simulink model "Noa_Nofusion_angle"  (R2020b)
settings: Solver=FixedStepDiscrete  StartTime=0.0  StopTime=Inf  FixedStep=0.01  RelTol=1e-3
PostLoadFcn:
  | if any(exist('dsrtsu_mdlpostloadfcn', 'file') ~= 0), dsrtsu_mdlpostloadfcn('Execute', bdroot); end
InitFcn:
  | , if any(exist('rtifpga_mdlclblib', 'file') ~= 0), rtifpga_mdlclblib('Init', bdroot); end,
  | , if any(exist('dsmpb_private', 'file') ~= 0), dsmpb_private('dsmpb_mdlclblib', 'Init', bdroot); end,
undefined symbols (not defined in the file): ACC_TimeGap_DecSetSwt, ACC_TimeGap_IncSetSwt, AccelPedalPosn, AccelPedalPosnVldty, AccelPedlPosnDiagc, AccPedalOverride, ACU_ShiftInProgress, ADAS_Posn_CurLane, AESSwtReq, ALC_SwtReq, BrkPedalSts, CC_ACC_CANCEL_OFFSwt, CC_ACC_CRUISE_OFFSwt, CC_ACC_DecSetSpd_SetSwt, CC_ACC_IncSetSpd_ResuSwt, CC_ACCSwtErr, CharSpd_ms, CSA_NODE, CURRENT_GEAR, CurrentGearValid, DiscIntNeverNeededParam, DrvDoorSts, DrvSBR, DrvTrqReqOvld, ECMACCInterface, ECMRespACC, ELKSwtReq, EngLimpHomeSts, EngSpd, EngState, EngState_PHEV, EngTrqMaxActSpd, EngTrqMinAct, EPS_DrvInpTrqVal_HighReslolution, EPS_FailSts, EPS_LKATorqOvrlDlvd, EPS_LKATorqOvrlDlvdVld, EPS_LKATrqOvlDlvdSts, EPS_SteerMod, EPS_TrqSnsrSts, EQ4_APPINFO, EQ4_LA_ELEM, EQ4_LA_HDR, EQ4_LAP_ELEM, EQ4_LAP_HDR, EQ4_LH_ELEM, EQ4_LH_HDR, EQ4_LRE_ELEM, EQ4_LRE_HDR, ESS_PedSwtReq, ESS_VehSwtReq, FFogLmpSts_F_Pbox, FLWheelDriveDirection, FLWheelSpd, FrntWiprSwtSts, FrntWshrSwtSts, FRWheelDriveDirection, FRWheelSpd, HazardLmpSwtSts, HCU_AccelPedalPosn_Diag ... (+151)
libraries: simulink x138, dsmpblib x33, canfdmsglib x10
(part 13 of 17)

== system Noa_Nofusion_angle/TOS/Subsystem1/ACCOSM/ObjMatrixTransit/Subsystem/For Each Subsystem ==
  <EQ4_OBJ_ELEM> : Inport  Partition=on  PartitionDimension=1  PartitionWidth=1  PartitionOffset=0
  Bus Selector : BusSelector  OutputSignals=OBJ_ID,OBJ_Existence_Probability,OBJ_Object_Class,OBJ_Width,OBJ_Long_Distance,OBJ_Lat_Distance,OBJ_Abs_Long_Acc,OBJ_Abs_Long_Velocity,OBJ_Abs_Lat_Velocity,OBJ_Brake_Light,OBJ_Object_Age,OBJ_Motion_Status,OBJ_Motion_Category,OBJ_Motion_Orientation
  For Each : ForEach  DisableCoverage=on
  id : Outport  ConcatenationDimension=1
  confidence : Outport  Port=2  ConcatenationDimension=1
  classification : Outport  Port=3  ConcatenationDimension=1
  width : Outport  Port=4  ConcatenationDimension=1
  LongDis : Outport  Port=5  ConcatenationDimension=1
  LatDis : Outport  Port=6  ConcatenationDimension=1
  AbsLongAcc : Outport  Port=7  ConcatenationDimension=1
  AbsLongVel : Outport  Port=8  ConcatenationDimension=1
  AbsLatVel : Outport  Port=9  ConcatenationDimension=1
  BrakeLight : Outport  Port=10  ConcatenationDimension=1
  Age : Outport  Port=11  ConcatenationDimension=1
  motionSts : Outport  Port=12  ConcatenationDimension=1
  motionCategory : Outport  Port=13  ConcatenationDimension=1
  motionOrientation : Outport  Port=14  ConcatenationDimension=1
  wires:
  <EQ4_OBJ_ELEM>/1 -> Bus Selector/1
  Bus Selector/12 -> motionSts/1  "<OBJ_Motion_Status>"
  Bus Selector/6 -> LatDis/1  "<OBJ_Lat_Distance>"
  Bus Selector/9 -> AbsLatVel/1  "<OBJ_Abs_Lat_Velocity>"
  Bus Selector/7 -> AbsLongAcc/1  "<OBJ_Abs_Long_Acc>"
  Bus Selector/1 -> id/1  "<OBJ_ID>"
  Bus Selector/2 -> confidence/1  "<OBJ_Existence_Probability>"
  Bus Selector/10 -> BrakeLight/1  "<OBJ_Brake_Light>"
  Bus Selector/8 -> AbsLongVel/1  "<OBJ_Abs_Long_Velocity>"
  Bus Selector/5 -> LongDis/1  "<OBJ_Long_Distance>"
  Bus Selector/11 -> Age/1  "<OBJ_Object_Age>"
  Bus Selector/4 -> width/1  "<OBJ_Width>"
  Bus Selector/14 -> motionOrientation/1  "<OBJ_Motion_Orientation>"
  Bus Selector/3 -> classification/1  "<OBJ_Object_Class>"
  Bus Selector/13 -> motionCategory/1  "<OBJ_Motion_Category>"

== system Noa_Nofusion_angle/TOS/Subsystem1/ACCOSM/ObjMatrixTransit/Subsystem/For Iterator Subsystem ==
  <EQ4_OBJ_ELEM> : Inport
  Bus Selector : BusSelector  OutputSignals=OBJ_ID,OBJ_Existence_Probability,OBJ_Object_Class,OBJ_Width,OBJ_Long_Distance,OBJ_Lat_Distance,OBJ_Abs_Long_Acc,OBJ_Abs_Long_Velocity,OBJ_Abs_Lat_Velocity,OBJ_Brake_Light,OBJ_Object_Age,OBJ_Motion_Status,OBJ_Motion_Category,OBJ_Motion_Orientation
  For Iterator : ForIterator  IterationLimit=20
  Selector : Selector  InputPortWidth=20  IndexOptions=Index vector (port)  Indices=[1 3]  OutputSizes=1
  id : Outport
  confidence : Outport  Port=2
  classification : Outport  Port=3
  width : Outport  Port=4
  LongDis : Outport  Port=5
  LatDis : Outport  Port=6
  AbsLongAcc : Outport  Port=7
  AbsLongVel : Outport  Port=8
  AbsLatVel : Outport  Port=9
  BrakeLight : Outport  Port=10
  Age : Outport  Port=11
  motionSts : Outport  Port=12
  motionCategory : Outport  Port=13
  motionOrientation : Outport  Port=14
  wires:
  <EQ4_OBJ_ELEM>/1 -> Selector/1
  For Iterator/1 -> Selector/2
  Selector/1 -> Bus Selector/1
  Bus Selector/1 -> id/1  "<OBJ_ID>"
  Bus Selector/2 -> confidence/1  "<OBJ_Existence_Probability>"
  Bus Selector/3 -> classification/1  "<OBJ_Object_Class>"
  Bus Selector/4 -> width/1  "<OBJ_Width>"
  Bus Selector/5 -> LongDis/1  "<OBJ_Long_Distance>"
  Bus Selector/6 -> LatDis/1  "<OBJ_Lat_Distance>"
  Bus Selector/7 -> AbsLongAcc/1  "<OBJ_Abs_Long_Acc>"
  Bus Selector/8 -> AbsLongVel/1  "<OBJ_Abs_Long_Velocity>"
  Bus Selector/9 -> AbsLatVel/1  "<OBJ_Abs_Lat_Velocity>"
  Bus Selector/10 -> BrakeLight/1  "<OBJ_Brake_Light>"
  Bus Selector/11 -> Age/1  "<OBJ_Object_Age>"
  Bus Selector/12 -> motionSts/1  "<OBJ_Motion_Status>"
  Bus Selector/13 -> motionCategory/1  "<OBJ_Motion_Category>"
  Bus Selector/14 -> motionOrientation/1  "<OBJ_Motion_Orientation>"

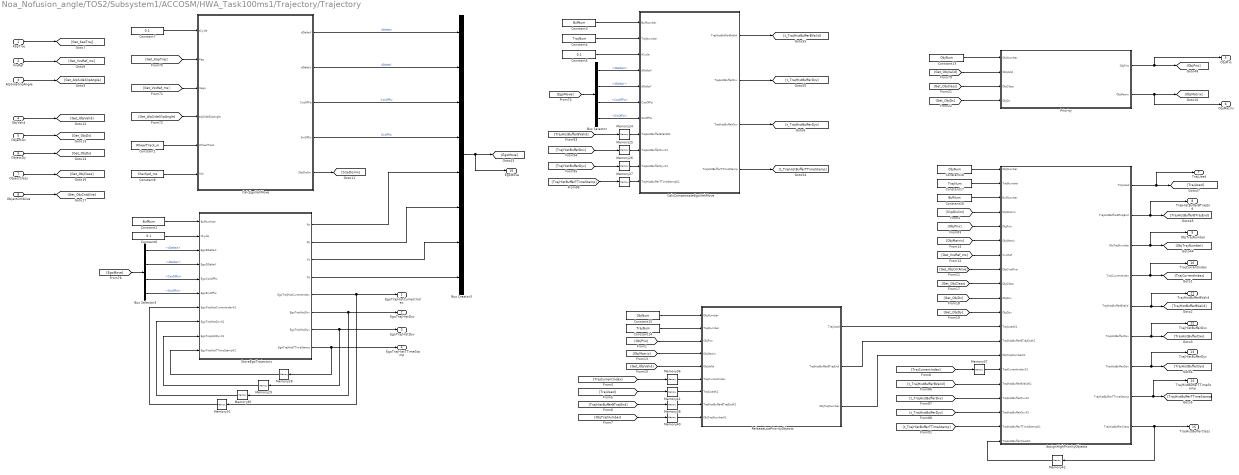
== system Noa_Nofusion_angle/TOS2/Subsystem1/ACCOSM/HWA_Task100ms1/Trajectory/Trajectory ==
  KapTraj : Inport
  VxvRef : Inport  Port=2
  AlpSideSlipAngle : Inport  Port=3
  ObjValid : Inport  Port=4
  ObjectDx : Inport  Port=5
  ObjectDy : Inport  Port=6
  ObjectClass : Inport  Port=7
  ObjectCntAlive : Inport  Port=8
  AssignHighPriorityObjects : MATLAB Function  TreatAsAtomicUnit=on
  Bus Creator3 : BusCreator  Inputs=8
  Bus Selector : BusSelector  OutputSignals=dDeltaX,dDeltaY,CosOfPsi,SinOfPsi
  Bus Selector3 : BusSelector  OutputSignals=dDeltaX,dDeltaY,CosOfPsi,SinOfPsi
  CalcCompensateEgoVehMove : MATLAB Function  TreatAsAtomicUnit=on
  CalcEgoVehMove : MATLAB Function  TreatAsAtomicUnit=on
  Constant1 : Constant  Value=WheelTrack_m  OutDataTypeStr=single
  Constant13 : Constant  Value=ObjNum  OutDataTypeStr=uint8
  Constant14 : Constant  Value=TrajNum  OutDataTypeStr=uint8
  Constant15 : Constant  Value=ObjNum  OutDataTypeStr=uint8
  Constant16 : Constant  Value=BufNum  OutDataTypeStr=uint8
  Constant17 : Constant  Value=TrajNum  OutDataTypeStr=uint8
  Constant18 : Constant  Value=ObjNum  OutDataTypeStr=uint8
  Constant2 : Constant  Value=BufNum  OutDataTypeStr=uint8
  Constant3 : Constant  Value=BufNum  OutDataTypeStr=uint8
  Constant4 : Constant  Value=TrajNum  OutDataTypeStr=uint8
  Constant5 : Constant  Value=0.1  OutDataTypeStr=single
  Constant6 : Constant  Value=0.1  OutDataTypeStr=single
  Constant7 : Constant  Value=0.1  OutDataTypeStr=single
  Constant8 : Constant  Value=CharSpd_ms  OutDataTypeStr=single
  Memory{24..26,42} (4 alike) : Memory  InitialCondition=zeros(TrajNum,BufNum)  InheritSampleTime=on
  Memory27 : Memory  InitialCondition=32*ones(TrajNum,BufNum)  InheritSampleTime=on
  Memory28 : Memory  InitialCondition=32*ones(BufNum,1)  InheritSampleTime=on
  Memory29 : Memory  InitialCondition=zeros(BufNum,1)  InheritSampleTime=on
  Memory30 : Memory  InitialCondition=zeros(BufNum,1)  InheritSampleTime=on
  Memory31 : Memory  InitialCondition=1  InheritSampleTime=on
  Memory36 : Memory  InitialCondition=ones(TrajNum,1)  InheritSampleTime=on
  Memory37 : Memory  InitialCondition=ones(TrajNum,1)  InheritSampleTime=on
  Memory38 : Memory  InitialCondition=ones(TrajNum,BufNum)  InheritSampleTime=on
  Memory40 : Memory  InitialCondition=255*ones(ObjNum,1)  InheritSampleTime=on
  Memory41 : Memory  InitialCondition=zeros(TrajNum,1)  InheritSampleTime=on
  Priority : MATLAB Function  TreatAsAtomicUnit=on
  ReleaseLowPriorityObjects : MATLAB Function  TreatAsAtomicUnit=on
  StoreEgoTrajectory : MATLAB Function  TreatAsAtomicUnit=on
  EgoTrajHistCurrentIndex : Outport
  EgoTrajHistDxv : Outport  Port=2
  EgoTrajHistDyv : Outport  Port=3
  EgoTrajHistTTimeStamp : Outport  Port=4
  ObjPrio : Outport  Port=5
  ObjMatrix : Outport  Port=6
  TrajUsed : Outport  Port=7
  TrajHistBufferBTrajEnd : Outport  Port=8
  ObjTrajNumber : Outport  Port=9
  TrajCurrentIndex : Outport  Port=10
  TrajHistBufferBValid : Outport  Port=11
  TrajHistBufferDxv : Outport  Port=12
  TrajHistBufferDyv : Outport  Port=13
  TrajHistBufferTTimeStamp : Outport  Port=14
  TrajHistBufferClass : Outport  Port=15
  EgoMove : Outport  Port=16
  wires:
  Constant7/1 -> CalcEgoVehMove/1(tCycle)
  [Get_VxvRef_ms] -> CalcEgoVehMove/3(Vego)
  [Get_AlpSideSlipAngle] -> CalcEgoVehMove/4(alpSideSlipAngle)
  [Get_KapTraj] -> CalcEgoVehMove/2(Kap)
  Constant5/1 -> CalcCompensateEgoVehMove/3(tCycle)
  Memory24/1 -> CalcCompensateEgoVehMove/8(TrajHistBufferBValidK1)
  Memory25/1 -> CalcCompensateEgoVehMove/9(TrajHistBufferDxvK1)
  Memory26/1 -> CalcCompensateEgoVehMove/10(TrajHistBufferDyvK1)
  Memory27/1 -> CalcCompensateEgoVehMove/11(TrajHistBufferTTimeStampK1)
  [EgoMove] -> Bus Selector/1
  Bus Selector/1 -> CalcCompensateEgoVehMove/4(dDeltaX)  "<dDeltaX>"
  Bus Selector/2 -> CalcCompensateEgoVehMove/5(dDeltaY)  "<dDeltaY>"
  Bus Selector/3 -> CalcCompensateEgoVehMove/6(CosOfPsi)  "<CosOfPsi>"
  Bus Selector/4 -> CalcCompensateEgoVehMove/7(SinOfPsi)  "<SinOfPsi>"
  [EgoMove] -> Bus Selector3/1
  [Get_ObjDx] -> Priority/4(ObjDx)
  [Get_ObjClass] -> Priority/3(ObjClass)
  [Get_ObjValid] -> Priority/2(ObjValid)
  ReleaseLowPriorityObjects/2(TrajHistBufferBTrajEnd) -> AssignHighPriorityObjects/13(TrajHistBufferBTrajEndK1)
  ReleaseLowPriorityObjects/1(TrajUsed) -> AssignHighPriorityObjects/12(TrajUsedK1)
  AssignHighPriorityObjects/3(ObjTrajNumber) -> ObjTrajNumber/1, [ObjTrajNumber]
  ReleaseLowPriorityObjects/3(ObjTrajNumber) -> AssignHighPriorityObjects/14(ObjTrajNumberK1)
  AssignHighPriorityObjects/1(TrajUsed) -> TrajUsed/1, [TrajUsed]
  AssignHighPriorityObjects/2(TrajHistBufferBTrajEnd) -> TrajHistBufferBTrajEnd/1, [TrajHistBufferBTrajEnd]
  AssignHighPriorityObjects/9(TrajHistBufferClass) -> Memory42/1, TrajHistBufferClass/1
  [ObjPrio] -> AssignHighPriorityObjects/5(ObjPrio)
  CalcCompensateEgoVehMove/1(TrajHistBufferBValid) -> [t_TrajHistBufferBValid]
  [t_TrajHistBufferBValid] -> AssignHighPriorityObjects/16(TrajHistBufferBValidK1)
  CalcCompensateEgoVehMove/2(TrajHistBufferDxv) -> [t_TrajHistBufferDxv]
  [t_TrajHistBufferDxv] -> AssignHighPriorityObjects/17(TrajHistBufferDxvK1)
  [t_TrajHistBufferDyv] -> AssignHighPriorityObjects/18(TrajHistBufferDyvK1)
  CalcCompensateEgoVehMove/4(TrajHistBufferTTimeStamp) -> [t_TrajHistBufferTTimeStamp]
  [t_TrajHistBufferTTimeStamp] -> AssignHighPriorityObjects/19(TrajHistBufferTTimeStampK1)
  Memory36/1 -> ReleaseLowPriorityObjects/6(TrajCurrentIndex)
  Memory37/1 -> AssignHighPriorityObjects/15(TrajCurrentIndexK1)
  Memory38/1 -> ReleaseLowPriorityObjects/8(TrajHistBufferBTrajEndK1)
  Memory40/1 -> ReleaseLowPriorityObjects/9(ObjTrajNumberK1)
  Memory41/1 -> ReleaseLowPriorityObjects/7(TrajUsedK1)
  Memory42/1 -> AssignHighPriorityObjects/20(TrajHistBufferClassK1)
  [TrajUsed] -> Memory41/1
  [ObjTrajNumber] -> Memory40/1
  [TrajHistBufferBTrajEnd] -> Memory38/1
  [ObjPrio] -> ReleaseLowPriorityObjects/3(ObjPrio)
  [Get_ObjValid] -> ReleaseLowPriorityObjects/5(ObjValid)
  AssignHighPriorityObjects/5(TrajHistBufferBValid) -> TrajHistBufferBValid/1, [TrajHistBufferBValid]
  AssignHighPriorityObjects/7(TrajHistBufferDyv) -> TrajHistBufferDyv/1, [TrajHistBufferDyv]
  AssignHighPriorityObjects/6(TrajHistBufferDxv) -> TrajHistBufferDxv/1, [TrajHistBufferDxv]
  [TrajCurrentIndex] -> Memory36/1
  [TrajCurrentIndex] -> Memory37/1
  [Get_VxvRef_ms] -> AssignHighPriorityObjects/7(VxvRef)
  [Get_ObjClass] -> AssignHighPriorityObjects/9(ObjClass)
  [Get_ObjDx] -> AssignHighPriorityObjects/10(ObjDxv)
  AssignHighPriorityObjects/4(TrajCurrentIndex) -> TrajCurrentIndex/1, [TrajCurrentIndex]
  [Get_ObjDy] -> AssignHighPriorityObjects/11(ObjDyv)
  [TrajHistBufferTTimeStamp] -> Memory27/1
  [TrajHistBufferDxv] -> Memory25/1
  [TrajHistBufferDyv] -> Memory26/1
  [TrajHistBufferBValid] -> Memory24/1
  [Get_ObjCntAlive] -> AssignHighPriorityObjects/8(ObjCntAlive)
  KapTraj/1 -> [Get_KapTraj]
  VxvRef/1 -> [Get_VxvRef_ms]
  AlpSideSlipAngle/1 -> [Get_AlpSideSlipAngle]
  Constant3/1 -> CalcCompensateEgoVehMove/1(BufNumber)
  Constant4/1 -> CalcCompensateEgoVehMove/2(TrajNumber)
  Constant13/1 -> Priority/1(ObjNumber)
  Constant15/1 -> ReleaseLowPriorityObjects/1(ObjNumber)
  Constant14/1 -> ReleaseLowPriorityObjects/2(TrajNumber)
  Constant18/1 -> AssignHighPriorityObjects/1(ObjNumber)
  Constant17/1 -> AssignHighPriorityObjects/2(TrajNumber)
  Constant16/1 -> AssignHighPriorityObjects/3(BufNumber)
  [ObjMatrix] -> ReleaseLowPriorityObjects/4(ObjMatrix)
  [ObjMatrix] -> AssignHighPriorityObjects/6(ObjMatrix)
  Constant2/1 -> StoreEgoTrajectory/1(BufNumber)
  Constant6/1 -> StoreEgoTrajectory/2(tCycle)
  StoreEgoTrajectory/7(EgoTrajHistDyv) -> EgoTrajHistDyv/1, Memory29/1
  Memory28/1 -> StoreEgoTrajectory/10(EgoTrajHistTTimeStampK1)
  Memory29/1 -> StoreEgoTrajectory/9(EgoTrajHistDyvK1)
  StoreEgoTrajectory/6(EgoTrajHistDxv) -> EgoTrajHistDxv/1, Memory30/1
  Memory30/1 -> StoreEgoTrajectory/8(EgoTrajHistDxvK1)
  StoreEgoTrajectory/5(EgoTrajHistCurrentIndex) -> EgoTrajHistCurrentIndex/1, Memory31/1
  Memory31/1 -> StoreEgoTrajectory/7(EgoTrajHistCurrentIndexK1)
  StoreEgoTrajectory/8(EgoTrajHistTTimeStamp) -> EgoTrajHistTTimeStamp/1, Memory28/1
  Bus Selector3/3 -> StoreEgoTrajectory/5(EgoCosOfPsi)  "<CosOfPsi>"
  Bus Selector3/2 -> StoreEgoTrajectory/4(EgoDDeltaY)  "<dDeltaY>"
  Bus Selector3/4 -> StoreEgoTrajectory/6(EgoSinOfPsi)  "<SinOfPsi>"
  Bus Selector3/1 -> StoreEgoTrajectory/3(EgoDDeltaX)  "<dDeltaX>"
  AssignHighPriorityObjects/8(TrajHistBufferTTimeStamp) -> TrajHistBufferTTimeStamp/1, [TrajHistBufferTTimeStamp]
  ObjValid/1 -> [Get_ObjValid]
  ObjectDy/1 -> [Get_ObjDy]
  ObjectDx/1 -> [Get_ObjDx]
  ObjectClass/1 -> [Get_ObjClass]
  ObjectCntAlive/1 -> [Get_ObjCntAlive]
  CalcEgoVehMove/1(dDeltaX) -> Bus Creator3/1  "dDeltaX"
  CalcEgoVehMove/2(dDeltaY) -> Bus Creator3/2  "dDeltaY"
  CalcEgoVehMove/3(CosOfPsi) -> Bus Creator3/3  "CosOfPsi"
  CalcEgoVehMove/4(SinOfPsi) -> Bus Creator3/4  "SinOfPsi"
  Priority/1(ObjPrio) -> ObjPrio/1, [ObjPrio]
  Priority/2(ObjMatrix) -> [ObjMatrix], ObjMatrix/1
  CalcCompensateEgoVehMove/3(TrajHistBufferDyv) -> [t_TrajHistBufferDyv]
  Constant1/1 -> CalcEgoVehMove/5(WheelTrack)
  Constant8/1 -> CalcEgoVehMove/6(Vch)
  CalcEgoVehMove/5(SlipDislim) -> [SlipDislim]
  [SlipDislim] -> AssignHighPriorityObjects/4(SlipDisLim)
  Bus Creator3/1 -> EgoMove/1, [EgoMove]
  StoreEgoTrajectory/4(Pd) -> Bus Creator3/8
  StoreEgoTrajectory/3(Pc) -> Bus Creator3/7
  StoreEgoTrajectory/2(Pb) -> Bus Creator3/6
  StoreEgoTrajectory/1(Pa) -> Bus Creator3/5

== system Noa_Nofusion_angle/TOS2/Subsystem1/ACCOSM/ObjMatrixTransit/Subsystem/For Each Subsystem ==
  <EQ4_OBJ_ELEM> : Inport  Partition=on  PartitionDimension=1  PartitionWidth=1  PartitionOffset=0
  Bus Selector : BusSelector  OutputSignals=OBJ_ID,OBJ_Existence_Probability,OBJ_Object_Class,OBJ_Width,OBJ_Long_Distance,OBJ_Lat_Distance,OBJ_Abs_Long_Acc,OBJ_Abs_Long_Velocity,OBJ_Abs_Lat_Velocity,OBJ_Brake_Light,OBJ_Object_Age,OBJ_Motion_Status,OBJ_Motion_Category,OBJ_Motion_Orientation
  For Each : ForEach  DisableCoverage=on
  id : Outport  ConcatenationDimension=1
  confidence : Outport  Port=2  ConcatenationDimension=1
  classification : Outport  Port=3  ConcatenationDimension=1
  width : Outport  Port=4  ConcatenationDimension=1
  LongDis : Outport  Port=5  ConcatenationDimension=1
  LatDis : Outport  Port=6  ConcatenationDimension=1
  AbsLongAcc : Outport  Port=7  ConcatenationDimension=1
  AbsLongVel : Outport  Port=8  ConcatenationDimension=1
  AbsLatVel : Outport  Port=9  ConcatenationDimension=1
  BrakeLight : Outport  Port=10  ConcatenationDimension=1
  Age : Outport  Port=11  ConcatenationDimension=1
  motionSts : Outport  Port=12  ConcatenationDimension=1
  motionCategory : Outport  Port=13  ConcatenationDimension=1
  motionOrientation : Outport  Port=14  ConcatenationDimension=1
  wires:
  <EQ4_OBJ_ELEM>/1 -> Bus Selector/1
  Bus Selector/12 -> motionSts/1  "<OBJ_Motion_Status>"
  Bus Selector/6 -> LatDis/1  "<OBJ_Lat_Distance>"
  Bus Selector/9 -> AbsLatVel/1  "<OBJ_Abs_Lat_Velocity>"
  Bus Selector/7 -> AbsLongAcc/1  "<OBJ_Abs_Long_Acc>"
  Bus Selector/1 -> id/1  "<OBJ_ID>"
  Bus Selector/2 -> confidence/1  "<OBJ_Existence_Probability>"
  Bus Selector/10 -> BrakeLight/1  "<OBJ_Brake_Light>"
  Bus Selector/8 -> AbsLongVel/1  "<OBJ_Abs_Long_Velocity>"
  Bus Selector/5 -> LongDis/1  "<OBJ_Long_Distance>"
  Bus Selector/11 -> Age/1  "<OBJ_Object_Age>"
  Bus Selector/4 -> width/1  "<OBJ_Width>"
  Bus Selector/14 -> motionOrientation/1  "<OBJ_Motion_Orientation>"
  Bus Selector/3 -> classification/1  "<OBJ_Object_Class>"
  Bus Selector/13 -> motionCategory/1  "<OBJ_Motion_Category>"

== system Noa_Nofusion_angle/TOS2/Subsystem1/ACCOSM/ObjMatrixTransit/Subsystem/For Iterator Subsystem ==
  <EQ4_OBJ_ELEM> : Inport
  Bus Selector : BusSelector  OutputSignals=OBJ_ID,OBJ_Existence_Probability,OBJ_Object_Class,OBJ_Width,OBJ_Long_Distance,OBJ_Lat_Distance,OBJ_Abs_Long_Acc,OBJ_Abs_Long_Velocity,OBJ_Abs_Lat_Velocity,OBJ_Brake_Light,OBJ_Object_Age,OBJ_Motion_Status,OBJ_Motion_Category,OBJ_Motion_Orientation
  For Iterator : ForIterator  IterationLimit=20
  Selector : Selector  InputPortWidth=20  IndexOptions=Index vector (port)  Indices=[1 3]  OutputSizes=1
  id : Outport
  confidence : Outport  Port=2
  classification : Outport  Port=3
  width : Outport  Port=4
  LongDis : Outport  Port=5
  LatDis : Outport  Port=6
  AbsLongAcc : Outport  Port=7
  AbsLongVel : Outport  Port=8
  AbsLatVel : Outport  Port=9
  BrakeLight : Outport  Port=10
  Age : Outport  Port=11
  motionSts : Outport  Port=12
  motionCategory : Outport  Port=13
  motionOrientation : Outport  Port=14
  wires:
  <EQ4_OBJ_ELEM>/1 -> Selector/1
  For Iterator/1 -> Selector/2
  Selector/1 -> Bus Selector/1
  Bus Selector/1 -> id/1  "<OBJ_ID>"
  Bus Selector/2 -> confidence/1  "<OBJ_Existence_Probability>"
  Bus Selector/3 -> classification/1  "<OBJ_Object_Class>"
  Bus Selector/4 -> width/1  "<OBJ_Width>"
  Bus Selector/5 -> LongDis/1  "<OBJ_Long_Distance>"
  Bus Selector/6 -> LatDis/1  "<OBJ_Lat_Distance>"
  Bus Selector/7 -> AbsLongAcc/1  "<OBJ_Abs_Long_Acc>"
  Bus Selector/8 -> AbsLongVel/1  "<OBJ_Abs_Long_Velocity>"
  Bus Selector/9 -> AbsLatVel/1  "<OBJ_Abs_Lat_Velocity>"
  Bus Selector/10 -> BrakeLight/1  "<OBJ_Brake_Light>"
  Bus Selector/11 -> Age/1  "<OBJ_Object_Age>"
  Bus Selector/12 -> motionSts/1  "<OBJ_Motion_Status>"
  Bus Selector/13 -> motionCategory/1  "<OBJ_Motion_Category>"
  Bus Selector/14 -> motionOrientation/1  "<OBJ_Motion_Orientation>"

== matlab function Noa_Nofusion_angle/TOS2/Subsystem1/ACCOSM/HWA_Task100ms1/OTL1/P0TrajHistCalc1 ==
  data: P0TrajHistNum output uint8; P0TrajHistNum1 input uint8; P0TrajHistDxv1 input single; P0TrajHistDxv output single; P0TrajHistDyv1 input single; P0TrajHistDyv output single; LineValid output boolean; a output single; b output single; c output single; d output single; dxMin output single; dxMax output single
function [P0TrajHistNum,P0TrajHistDxv,P0TrajHistDyv,LineValid,a,b,c,d,dxMin,dxMax] = P0TrajHistMixCalc(...
    P0TrajHistNum1,P0TrajHistDxv1,P0TrajHistDyv1)

P0TrajHistDxv = single(zeros(48,1));
P0TrajHistDyv = single(zeros(48,1));
P0TrajHistNum = uint8(0);

if (P0TrajHistNum1>0)
    P0TrajHistDxv(1:P0TrajHistNum1) = P0TrajHistDxv1(1:P0TrajHistNum1);
    P0TrajHistDyv(1:P0TrajHistNum1) = P0TrajHistDyv1(1:P0TrajHistNum1);
    P0TrajHistNum = P0TrajHistNum1;
end

if P0TrajHistNum>=4
    dxMin = P0TrajHistDxv(P0TrajHistNum);
    dxMax = P0TrajHistDxv(1) + 6;
%     q2 = max(ceil(P0TrajHistNum/2),2);
%     q3 = max(ceil(P0TrajHistNum*3/4),3);
%     q4 = P0TrajHistNum;
%     MaX = [P0TrajHistDxv(1);P0TrajHistDxv(q2);P0TrajHistDxv(q3);P0TrajHistDxv(q4)];
%     MaY = [P0TrajHistDyv(1);P0TrajHistDyv(q2);P0TrajHistDyv(q3);P0TrajHistDyv(q4)];
%     [~,b,c,d] = pl(MaX,MaY);
    P = polyfit(P0TrajHistDxv(1:P0TrajHistNum),P0TrajHistDyv(1:P0TrajHistNum),2);
    b = P(1);
    c = P(2);
    d = P(3);

    a = single(0);
   LineValid = true;
   if dxMin>0.5
      LineValid = false; 
   end
else
   dxMin = single(0); 
   dxMax = single(0); 
   a = single(0);
   b = single(0);
   c = single(0);
   d = single(0);
   LineValid = false;
end

== matlab function Noa_Nofusion_angle/TOS2/Subsystem1/ACCOSM/HWA_Task100ms1/Plaus ==
  data: dxMaxFollow input single size=1; ObjValid input boolean size=15; ObjDx input single size=15; ObjVx input single size=15; ObjPlaus output single size=15; ObjOnLeft input single size=15; ObjPlausLeft output single size=15; ObjPlausRight output single size=15; ObjOnRight input single size=15; ObjDycHist input single size=15; ObjqDycHist input single size=15; ObjLpb input single size=15; ObjLpbLeft input single size=15; ObjLpbRight input single size=15; ObjPlausK1 input single size=15; ObjPlausLeftK1 input single size=15; ObjPlausRightK1 input single size=15
function [ObjPlaus,ObjPlausLeft,ObjPlausRight] = ...
    PlausCalc(dxMaxFollow,ObjValid,ObjDx,ObjVx,ObjOnLeft,ObjOnRight,ObjDycHist,ObjqDycHist,...
    ObjLpb,ObjLpbLeft,ObjLpbRight,ObjPlausK1,ObjPlausLeftK1,ObjPlausRightK1)

[ObjPlaus,ObjPlausLeft,ObjPlausRight] = ...
    PlausCalc(dxMaxFollow,ObjValid,ObjDx,ObjVx,ObjOnLeft,ObjOnRight,ObjDycHist,ObjqDycHist,...
    ObjLpb,ObjLpbLeft,ObjLpbRight,ObjPlausK1,ObjPlausLeftK1,ObjPlausRightK1);
end

== matlab function Noa_Nofusion_angle/TOS2/Subsystem1/ACCOSM/HWA_Task100ms1/Spw ==
  data: AlpSumSlideCurveness input single size=1; kapCourseErr input single size=1; ObjSpw output single size=15; ObjValid input boolean size=15; DycASI input single size=15; ObjDx input single size=15; ObjSpwLeft output single size=15; ObjSpwRight output single size=15; ObjOnLeft output; ObjOnRight output; ObjDyc input; ObjDycHist input; ObjqDycHist input; ObjDycASI output; ObjDyKapErr output
function [ObjSpw,ObjSpwLeft,ObjSpwRight,ObjOnLeft,ObjOnRight,ObjDycASI,ObjDyKapErr] = ...
    CalcSpw(AlpSumSlideCurveness,kapCourseErr,ObjValid,DycASI,ObjDx,ObjDyc,ObjDycHist,ObjqDycHist)
 
ObjSpw = single(zeros(15,1));
ObjSpwLeft = single(zeros(15,1));
ObjSpwRight = single(zeros(15,1));
ObjOnLeft = single(zeros(15,1));
ObjOnRight = single(zeros(15,1));
ObjDycASI = single(zeros(15,1));
ObjDyKapErr = single(zeros(15,1));
 
for i=1:15
    if ObjValid(i)
        t_dycASI = DycASI(i);
        t_kapErrMin = single(0.0002);
        t_kapErrCurvenessMax = single(0.0018);
        
        temp1 = min(AlpSumSlideCurveness,single(1));
        t_kapErrCurveness = t_kapErrCurvenessMax*temp1;
        t_kapErr = max(t_kapErrMin,max(kapCourseErr,t_kapErrCurveness));
        temp1 = min(ObjDx(i),single(80));
        t_DyKapErr = t_kapErr*temp1*temp1/2;
        ObjDyKapErr(i) = t_DyKapErr;
        
        %         t_dyHalfLane = 1.5;
        %         t_dy3halfLane = 5.25;
        
        if abs(t_dycASI)>=4.5
            t_spw = single(0);
            t_spwNeighbour = single(0);
        elseif abs(t_dycASI)>=3
            t_spw = single(0);
            t_dycToLane = abs(t_dycASI) - single(3);
            t_spwNeighbour = CalcSPW(t_dycToLane,single(3),t_DyKapErr);
        elseif abs(t_dycASI)>=1.5
            t_spw = single(0);
            t_spwNeighbour = CalcSPW(single(0),single(3),t_DyKapErr);
        else
            t_spwNeighbour = single(0);
            t_spw = CalcSPW(single(0),single(3),t_DyKapErr);
        end
        if t_dycASI>=0
            t_spwRight = single(0);
            t_spwLeft = t_spwNeighbour;
        else
            t_spwLeft = single(0);
            t_spwRight = t_spwNeighbour;
        end
        ObjSpw(i) = t_spw;
        ObjSpwLeft(i) = t_spwLeft;
        ObjSpwRight(i) = t_spwRight;
        % -------------------------------------------------------------------------
        
        temp1 = 0.5*ObjqDycHist(i);
        t_dycASI = ObjDyc(i)*(1-temp1) + ObjDycHist(i)*temp1;
        temp2 = single(1.5) + t_DyKapErr;
        temp3 = single(3) + t_DyKapErr;
        ObjDycASI(i) = t_dycASI;
        
        if t_dycASI>=0
            temp1 = max(single(1.5),min(temp3,t_dycASI)) - single(1.5);
            ObjOnLeft(i) = min(single(1),temp1/temp2);
        else
            temp1 = max(min(single(-1.5),t_dycASI),-temp3);
            temp1 = -temp1 - single(1.5);
            ObjOnRight(i) = min(single(1),temp1/temp2);
        end
    end
end
end
 
function t_spw = CalcSPW(absDyc,dyLaneWidth,dyKapErr)
temp3 = dyLaneWidth/2;
temp1 = temp3 - dyKapErr;
temp2 = temp3 + dyKapErr;
temp2 = min(temp2,dyLaneWidth);
 
if absDyc<=temp1
    t_spw = single(1);
elseif absDyc>=temp2
    t_spw = single(0);
else
    temp3 = temp2 - absDyc;
    temp4 = 2*dyKapErr;
    t_spw = temp3/temp4;
end
end

== matlab function Noa_Nofusion_angle/TOS2/Subsystem1/ACCOSM/HWA_Task100ms1/Std ==
  data: u input; y output
function y = fcn(u)

y = std(u);

== stateflow chart Noa_Nofusion_angle/Common/Subsystem7/DS/DriverSts_StateMachine ==
  state DriverSts [group]
    0x0:DriverUnbeliv
    0x1:DriverGood
    0x2:DriverLowDistractn
    0x3:DriverMidDistractn
    0x4:DriverHi1Distractn
    0x5:DriverHi2Distractn
    0x6:DriverLowDrowsiness
    0x7:DriverMidDrowsiness
    0x8:DriverHi1Drowsiness
    0x9:DriverHi2Drowsiness
  state DistractnSts [group]
    0x0:DMSNoDistractn
    0x1:DMSLowDistractn
    0x2:DMSMidDistractn
    0x3:DMSHi1Distractn
    0x4:DMSHi2Distractn
    0x5:DMSUnbelievDistractn
    DrowsnsSts
    0x0:DMSNoDrowsiness
    0x1:DMSLowDrowsiness
    0x2:DMSMidDrowsiness
    0x3:DMSHi1Drowsiness
    0x4:DMSHi2Drowsiness
    0x5:DMSUnbelievDrowsiness
  state Ini
    entry: DriverSts=DriverUnbeliv;
    DADistractnNoDistractn=0;
    DADrowsnsNoDrowsiness=0;
  state Unbelievable
    entry: DriverSts=DriverUnbeliv;
    DistractnSts=DMSUnbelievDistractn;
    DrowsnsSts=DMSUnbelievDrowsiness;
  state Good
    entry:DriverSts=DriverGood;
    DistractnSts=DMSNoDistractn;
    DrowsnsSts=DMSNoDrowsiness;
  state DDA
    state Distractn [parallel]
      settings: executionOrder=1
      state NoDis
        entry:DistractnSts=DMSNoDistractn;
        DADistractnNoDistractn=1;
        exit:DADistractnNoDistractn=0;
      state ExistDis
        state LowDis
          entry:DistractnSts=DMSLowDistractn;
        state MidDis
          entry:DistractnSts=DMSMidDistractn;
        state Hi1Dis
          entry:DistractnSts=DMSHi1Distractn;
        state Hi2Dis
          entry:DistractnSts=DMSHi2Distractn;
        LowDis -> (junction 143) [order 2] : [DSOther2Hi1Distractn]
        (junction 143) -> (junction 126)
        (default) -> (junction 137)
        (junction 137) -> LowDis [order 1] : [DSGoodUnbeliv2LowDistractn]
        (junction 146) -> LowDis
        (junction 147) -> (junction 146)
        (junction 137) -> (junction 142) [order 2]
        (junction 144) -> (junction 146) [order 1] : [DSMidHi1Hi22LowDistractn]
        (junction 124) -> (junction 147) [order 1] : [DSMidHi1Hi22LowDistractn]
        LowDis -> MidDis [order 1] : [DSLow2MidDistractn]
        MidDis -> LowDis [order 2] : [DSMidHi1Hi22LowDistractn]
        (junction 142) -> MidDis [order 1] : [DSGoodUnbeliv2MidDistractn]
        (junction 144) -> MidDis [order 2]
        (junction 124) -> (junction 144) [order 2]
        (junction 142) -> (junction 138) [order 2]
        Hi2Dis -> (junction 144) : [DSHi1Hi22MidDistractn||......
            | DSMidHi1Hi22LowDistractn]
        (junction 130) -> (junction 124)
        MidDis -> Hi1Dis [order 1] : [DSOther2Hi1Distractn]
        Hi1Dis -> MidDis [order 2] : [DSHi1Hi22MidDistractn]
        Hi1Dis -> Hi2Dis [order 1] : [DSOther2Hi2Distractn]
        (junction 138) -> Hi1Dis
        (junction 126) -> Hi1Dis
        Hi1Dis -> (junction 130) [order 3] : [DSHi1Hi22MidDistractn||......
            | DSMidHi1Hi22LowDistractn]
      (default) -> (junction 122)
      (junction 122) -> NoDis [order 2]
      (junction 122) -> ExistDis [order 1] : [DSGoodUnbeliv2LowDistractn||......
          | DSGoodUnbeliv2MidDistractn||......
          | DSOther2Hi1Distractn]
      NoDis -> ExistDis : [DSGoodUnbeliv2LowDistractn||......
          | DSGoodUnbeliv2MidDistractn||......
          | DSOther2Hi1Distractn]
      ExistDis -> NoDis : [DSMidHi1Hi22NoDistractn]
    state Drowsns [parallel]
      settings: executionOrder=2
      state NoDrow
        entry:DrowsnsSts=DMSNoDrowsiness;
        DADrowsnsNoDrowsiness=1;
        exit:DADrowsnsNoDrowsiness=0;
      state ExistDrow
        state LowDrow
          entry:DrowsnsSts=DMSLowDrowsiness;
        state MidDrow
          entry:DrowsnsSts=DMSMidDrowsiness;
        state Hi1Drow
          entry:DrowsnsSts=DMSHi1Drowsiness;
        state Hi2Drow
          entry:DrowsnsSts=DMSHi2Drowsiness;
        LowDrow -> (junction 58) [order 2] : [DSOther2Hi1Drowsns]
        (junction 58) -> (junction 46)
        (default) -> (junction 36)
        (junction 36) -> LowDrow [order 1] : [DSGoodUnbeliv2LowDrowsns]
        (junction 10) -> LowDrow
        (junction 74) -> (junction 10)
        (junction 36) -> (junction 42) [order 2]
        (junction 11) -> (junction 10) [order 1] : [DSMidHi1Hi22LowDrowsns]
        (junction 61) -> (junction 74) [order 1] : [DSMidHi1Hi22LowDrowsns]
        LowDrow -> MidDrow [order 1] : [DSLow2MidDrowsns]
        MidDrow -> LowDrow [order 2] : [DSMidHi1Hi22LowDrowsns]
        (junction 42) -> MidDrow [order 1] : [DSGoodUnbeliv2MidDrowsns]
        (junction 11) -> MidDrow [order 2]
        (junction 61) -> (junction 11) [order 2]
        (junction 42) -> (junction 59) [order 2]
        Hi2Drow -> (junction 11) : [DSMidHi1Hi22LowDrowsns||......
            | DSHi1Hi22MidDrowsns]
        (junction 39) -> (junction 61)
        MidDrow -> Hi1Drow [order 1] : [DSOther2Hi1Drowsns]
        Hi1Drow -> MidDrow [order 2] : [DSHi1Hi22MidDrowsns]
        Hi1Drow -> Hi2Drow [order 1] : [DSOther2Hi2Drowsns]
        (junction 59) -> Hi1Drow
        (junction 46) -> Hi1Drow
        Hi1Drow -> (junction 39) [order 3] : [DSMidHi1Hi22LowDrowsns||......
            | DSHi1Hi22MidDrowsns]
      (default) -> (junction 72)
      (junction 72) -> NoDrow [order 2]
      (junction 72) -> ExistDrow [order 1] : [DSGoodUnbeliv2LowDrowsns||......
          | DSGoodUnbeliv2MidDrowsns||......
          | DSOther2Hi1Drowsns]
      NoDrow -> ExistDrow : [DSGoodUnbeliv2LowDrowsns||......
          | DSGoodUnbeliv2MidDrowsns||......
          | DSOther2Hi1Drowsns]
      ExistDrow -> NoDrow : [DSMidHi1Hi22NoDrowsns]
    state Arbitrate [parallel]
      settings: executionOrder=3
      Arbitrate -> (junction 20)
      (junction 20) -> (junction 75) [order 1] : [DistractnSts<DrowsnsSts]
      (junction 75) -> (junction 45) [order 1] : [DrowsnsSts==DMSHi2Drowsiness]
          | {DriverSts=DriverHi2Drowsiness;}
      (junction 20) -> (junction 14) [order 2]
      (junction 75) -> (junction 54) [order 2]
      (junction 45) -> (junction 19)
      (junction 14) -> (junction 48) [order 1] : [DistractnSts==DMSHi2Distractn]
          | {DriverSts=DriverHi2Distractn;}
      (junction 54) -> (junction 19) [order 1] : [DrowsnsSts==DMSHi1Drowsiness]
          | {DriverSts=DriverHi1Drowsiness;}
      (junction 14) -> (junction 89) [order 2]
      (junction 48) -> (junction 1)
      (junction 54) -> (junction 4) [order 2]
      (junction 19) -> (junction 5)
      (junction 89) -> (junction 1) [order 1] : [DistractnSts==DMSHi1Distractn]
          | {DriverSts=DriverHi1Distractn;}
      (junction 4) -> (junction 5) [order 1] : [DrowsnsSts==DMSMidDrowsiness]
          | {DriverSts=DriverMidDrowsiness;}
      (junction 89) -> (junction 95) [order 2]
      (junction 1) -> (junction 105)
      (junction 4) -> (junction 97) [order 2] : {DriverSts=DriverLowDrowsiness;}
      (junction 5) -> (junction 102)
      (junction 95) -> (junction 105) [order 1] : [DistractnSts==DMSMidDistractn]
          | {DriverSts=DriverMidDistractn;}
      (junction 105) -> (junction 93)
      (junction 95) -> (junction 99) [order 2] : {DriverSts=DriverLowDistractn;}
      (junction 93) -> (junction 99)
      (junction 97) -> (junction 93)
      (junction 102) -> (junction 97)
      (junction 99) -> Arbitrate
  (default) -> Ini
  Ini -> Unbelievable
  Unbelievable -> Good [order 2] : [DSOther2Good]
  Good -> Unbelievable [order 1] : [DSOther2Unbeliv]
  Unbelievable -> DDA [order 1] : [(DSGoodUnbeliv2LowDistractn||......
      | DSGoodUnbeliv2MidDistractn||......
      | DSOther2Hi1Distractn||......
      | DSGoodUnbeliv2LowDrowsns||......
      | DSGoodUnbeliv2MidDrowsns||......
      | DSOther2Hi1Drowsns)&&......
      | DSUnbeliv2DDAEnable]
  DDA -> Unbelievable [order 1] : [DSOther2Unbeliv]
  DDA -> Good [order 2] : [DSOther2Good||(DADistractnNoDistractn&&DADrowsnsNoDrowsiness)]
  Good -> DDA [order 2] : [DSGoodUnbeliv2LowDistractn||......
      | DSGoodUnbeliv2MidDistractn||......
      | DSOther2Hi1Distractn||......
      | DSGoodUnbeliv2LowDrowsns||......
      | DSGoodUnbeliv2MidDrowsns||......
      | DSOther2Hi1Drowsns]
  data: DSOther2Good input; DSOther2Unbeliv input; DADistractnNoDistractn local uint8; DADrowsnsNoDrowsiness local uint8; DistractnSts output uint8 =uint8(0); DrowsnsSts output uint8 =uint8(0); DMSHi1Distractn local uint8 =uint8(3); DMSHi1Drowsiness local uint8 =uint8(3); DMSHi2Distractn local uint8 =uint8(4); DMSHi2Drowsiness local uint8 =uint8(4); DMSLowDistractn local uint8 =uint8(1); DMSLowDrowsiness local uint8 =uint8(1); DMSMidDistractn local uint8 =uint8(2); DMSMidDrowsiness local uint8 =uint8(2); DMSNoDistractn local uint8 =uint8(0); DMSNoDrowsiness local uint8 =uint8(0); DMSUnbelievDistractn local uint8 =uint8(5); DMSUnbelievDrowsiness local uint8 =uint8(5); DriverGood local uint8 =uint8(1); DriverHi1Distractn local uint8 =uint8(4); DriverHi1Drowsiness local uint8 =uint8(8); DriverHi2Distractn local uint8 =uint8(5); DriverHi2Drowsiness local uint8 =uint8(9); DriverLowDistractn local uint8 =uint8(2); DriverLowDrowsiness local uint8 =uint8(6); DriverMidDistractn local uint8 =uint8(3); DriverMidDrowsiness local uint8 =uint8(7); DriverSts output uint8; DriverUnbeliv local uint8 =uint8(0); DSGoodUnbeliv2LowDistractn input; DSMidHi1Hi22LowDistractn input; DSGoodUnbeliv2MidDistractn input; DSLow2MidDistractn input; DSHi1Hi22MidDistractn input; DSOther2Hi1Distractn input; DSOther2Hi2Distractn input; DSGoodUnbeliv2LowDrowsns input; DSMidHi1Hi22LowDrowsns input; DSGoodUnbeliv2MidDrowsns input; DSLow2MidDrowsns input; DSHi1Hi22MidDrowsns input; DSOther2Hi1Drowsns input; DSOther2Hi2Drowsns input; DSMidHi1Hi22NoDistractn input; DSMidHi1Hi22NoDrowsns input; DSUnbeliv2DDAEnable input

== matlab function Noa_Nofusion_angle/TOS2/Subsystem1/ACCOSM/HWA_Task100ms1/TargetBrake ==
  data: ID input uint8; VxG input; VyG input; TargetBrake_b output boolean; TargetVxG output; BrakeLightIndic input uint8 size=15; TargetVyG output
function [TargetBrake_b,TargetVxG,TargetVyG] = fcn(ID,VxG,VyG,BrakeLightIndic)
%#codegen
TargetBrake_b = false;
TargetVxG = single(0);
TargetVyG = single(0);

if (ID>0)&&(ID<100)
    if BrakeLightIndic(ID)==2
        TargetBrake_b = true;
    end
    TargetVxG = VxG(ID);
    TargetVyG = VyG(ID);
end

== matlab function Noa_Nofusion_angle/TOS2/Subsystem1/ACCOSM/HWA_Task100ms1/TargetSelect ==
  data: ACCmode input uint8 size=1; P0ID output uint8 size=1; vRef input single size=1; Valid input boolean size=15; Range input single size=15; Vr input single size=15; Dx input single size=15; Dy input single size=15; ArG input single size=15; Dyc input single size=15; Vyc input single size=15; Cnt input; plaus input single size=15; wCutIn input single size=15; spw input single size=15; spwLeft input single size=15; spwRight input single size=15; ReID input uint8 size=1; ReRange input single size=1; ReArG input single size=1; ReDx input single size=1; ReDy input single size=1; ReVx input single size=1; ReCutIn_b input boolean size=1; ReDyc input single size=1; ReVyc input single size=1; TargetLost_b input; tTargetLost input single size=1; dyLaneWidth input single size=1; Classfication input uint8 size=15; MoveSts input uint8 size=15; TarLimDx input single size=1; TarLimS0Dx input; TargetExistK1 input boolean size=1; P2ID output uint8 size=1; P3ID output uint8 size=1; P0Range output single size=1; P2Range output single size=1; P3Range output single size=1; P0Vr output single size=1; P2Vr output single size=1; P3Vr output single size=1; P0ArG output single size=1; P2ArG output single size=1; P3ArG output single size=1; P0Dx output single size=1; P2Dx output single size=1; P3Dx output single size=1; P0Dy output single size=1; P2Dy output single size=1; P3Dy output single size=1; TargetCutIn_b output boolean size=1; P0Dyc output single size=1; P0Vyc output single size=1; TargetExist output boolean size=1; TargetReplacedCntK1 input uint8; TargetReplacedCnt output uint8
function [P0ID,P2ID,P3ID,P0Range,P2Range,P3Range,P0Vr,P2Vr,P3Vr,P0ArG,P2ArG,P3ArG,...
    P0Dx,P2Dx,P3Dx,P0Dy,P2Dy,P3Dy,TargetCutIn_b,P0Dyc,P0Vyc,TargetExist,TargetReplacedCnt] = ...
    ATS(ACCmode,vRef,Valid,Range,Vr,Dx,Dy,ArG,Dyc,Vyc,Cnt,plaus,wCutIn,spw,spwLeft,spwRight,...
    ReID,ReRange,ReArG,ReDx,ReDy,ReVx,ReCutIn_b,ReDyc,ReVyc,TargetLost_b,tTargetLost,dyLaneWidth,...
    Classfication,MoveSts,TarLimDx,TarLimS0Dx,TargetExistK1,TargetReplacedCntK1)

% #codegen
% ACCMode
% 0x00:OFF mode
% 0x01:Passive mode(Reject)
% 0x02:Passive mode(Stand-by)
% 0x03:Active-Control mode
% 0x04:Brake-only mode
% 0x05:Override
% 0x06:Standstill
% 0x07:Failure mode
% 0x08~0x1F:Reserved

P0ID = uint8(0);
P2ID = uint8(0);
P3ID = uint8(0);
P0Range = single(255);
P2Range = single(255);
P3Range = single(255);
P0Vr = single(0);
P2Vr = single(0);
P3Vr = single(0);
P0ArG = single(0);
P2ArG = single(0);
P3ArG = single(0);
P0Dx = single(255);
P2Dx = single(255);
P3Dx = single(255);
P0Dy = single(0);
P2Dy = single(0);
P3Dy = single(0);
TargetExist = false;
TargetCutIn_b = false;
P0Dyc = single(0);
P0Vyc = single(0);

DycOffset = interpolate(single(50),single(0.35),single(80),single(0.6),ReDx);

if TargetLost_b
   TargetReplacedCnt = uint8(0);
else
   TargetReplacedCnt = min(uint8(255),TargetReplacedCntK1 + uint8(1));
end

if (ACCmode==1)||(ACCmode==2)||(ACCmode==3)||(ACCmode==4)||(ACCmode==5)||(ACCmode==6)||(ACCmode==9)
    if TargetExistK1==false   % first select target
        for i=1:15
            if (Valid(i)==1)&&(Cnt(i)>=3)&&...
                    (((vRef<=15.83)&&((MoveSts(i)==1)||(MoveSts(i)==2)||(MoveSts(i)==3)))||...
                    ((vRef>15.83)&&((MoveSts(i)==2)||(MoveSts(i)==3))))
                if (Classfication(i)==1)||(Classfication(i)==2)||(Classfication(i)==3)||(Classfication(i)==9)
                    if ((Range(i)<=TarLimS0Dx)&&(MoveSts(i)==1))||((Range(i)<=TarLimDx)&&((MoveSts(i)==2)||(MoveSts(i)==3)))
                        if (plaus(i)>=0.4)||((wCutIn(i)>0.7)&&(spw(i)>=0.8))||((spw(i)>0.95)&&(Range(i)<1.5*vRef))         % Need Check!
                            if Range(i)<P0Range
                                P0ID = uint8(i);
                                P0Range = Range(i);
                            end
                        else
                            if spwLeft(i)>0.2
                                if Range(i)<P2Range
                                    P2ID = uint8(i);
                                    P2Range = Range(i);
                                end
                            end
                            if spwRight(i)>0.2
                                if Range(i)<P3Range
                                    P3ID = uint8(i);
                                    P3Range = Range(i);
                                end
                            end
                        end
                    end
                end
            end
        end
    else
        k = ReID;
        if k<100        % No Target Lost!!!
            if (Valid(k)==0)
                for i=1:15
                    if (Valid(i)==1)&&...
                            (((vRef<=15.83)&&((MoveSts(i)==1)||(MoveSts(i)==2)||(MoveSts(i)==3)))||...
                            ((vRef>15.83)&&((MoveSts(i)==2)||(MoveSts(i)==3))))
                        if (Classfication(i)==1)||(Classfication(i)==2)||(Classfication(i)==3)||(Classfication(i)==9)
                            if ((Range(i)<=TarLimS0Dx)&&(MoveSts(i)==1))||((Range(i)<=TarLimDx)&&((MoveSts(i)==2)||(MoveSts(i)==3)))
                                if (plaus(i)>=0.4)||((wCutIn(i)>0.7)&&(spw(i)>=0.8))||((spw(i)>0.95)&&(Range(i)<1.5*vRef))
                                    if Range(i)<P0Range
                                        P0ID = uint8(i);
                                        P0Range = Range(i);
                                    end
                                else
                                    if spwLeft(i)>0.2
                                        if Range(i)<P2Range
                                            P2ID = uint8(i);
                                            P2Range = Range(i);
                                        end
                                    end
                                    if spwRight(i)>0.2
                                        if Range(i)<P3Range
                                            P3ID = uint8(i);
                                            P3Range = Range(i);
                                        end
                                    end
                                end
                            end
                        end
                    end
                end
            else
                temp = interpolate(single(5),single(10),single(30),single(20),vRef);
                
                if TargetReplacedCnt>4   % no Target lost  Or  After Target 4  cnt!
                    if ((Range(k)<=(TarLimS0Dx+temp))&&(MoveSts(k)==1))||((Range(k)<=(TarLimDx+temp))&&((MoveSts(k)==2)||(MoveSts(k)==3)))
                        if (plaus(k)>=0.2)||((wCutIn(k)>0.6)&&(spw(k)>=0.4))||(spw(k)>0.6)
                            if Range(k)<P0Range
                                P0ID = uint8(k);
                                P0Range = Range(k);
                            end
                        else
                            if spwLeft(k)>0.2
                                if Range(k)<P2Range
                                    P2ID = uint8(k);
                                    P2Range = Range(k);
                                end
                            end
                            if spwLeft(k)>0.2
                                if Range(k)<P3Range
                                    P3ID = uint8(k);
                                    P3Range = Range(k);
                                end
                            end
                        end
                    end
                else  % After lost Target  Replaced  1\2\3 Cnt ！
                    if (Range(k)<(TarLimDx+temp))
                        if (spw(k)>=0.8)||((wCutIn(k)>0.7)&&(spw(k)>=0.4))
                            if Range(k)<P0Range
                                P0ID = uint8(k);
                                P0Range = Range(k);
                            end
                        else
                            if spwLeft(k)>0.2
                                if Range(k)<P2Range
                                    P2ID = uint8(k);
                                    P2Range = Range(k);
                                end
                            end
                            if spwLeft(k)>0.2
                                if Range(k)<P3Range
                                    P3ID = uint8(k);
                                    P3Range = Range(k);
                                end
                            end
                        end
                    end
                end %  After lost Target Replaced  //end 
                for i=1:15
                    if (i~=k)&&(Valid(i)==1)&&...
                            (((vRef<=15.83)&&((MoveSts(i)==1)||(MoveSts(i)==2)||(MoveSts(i)==3)))||...
                            ((vRef>15.83)&&((MoveSts(i)==2)||(MoveSts(i)==3))))
                        if (Classfication(i)==1)||(Classfication(i)==2)||(Classfication(i)==3)||(Classfication(i)==9)
                            if ((Range(i)<=TarLimS0Dx)&&(MoveSts(i)==1))||((Range(i)<=TarLimDx)&&((MoveSts(i)==2)||(MoveSts(i)==3)))
                                if (plaus(i)>=0.4)||((wCutIn(i)>0.7)&&(spw(i)>=0.8))||((spw(i)>0.95)&&(Range(i)<1.5*vRef))
                                    if Range(i)<P0Range
                                        P0ID = uint8(i);
                                        P0Range = Range(i);
                                    end
                                else
                                    if spwLeft(i)>0.2
                                        if Range(i)<P2Range
                                            P2ID = uint8(i);
                                            P2Range = Range(i);
                                        end
                                    end
                                    if spwRight(i)>0.2
                                        if Range(i)<P3Range
                                            P3ID = uint8(i);
                                            P3Range = Range(i);
                                        end
                                    end
                                end
                            end
                        end
                    end
                end
            end
        else
            temp = interpolate(single(5),single(10),single(30),single(20),vRef);
            if (ReRange<(TarLimDx+temp))&&(tTargetLost<0.6)
                if (ReDyc<(DycOffset + dyLaneWidth))&&(ReDyc>(-dyLaneWidth - DycOffset))
                   P0ID = k;
                   P0Range = ReRange;
                end
            end
            for i=1:15
                if (Valid(i)==1)&&...
                        (((vRef<=15.83)&&((MoveSts(i)==1)||(MoveSts(i)==2)||(MoveSts(i)==3)))||...
                        ((vRef>15.83)&&((MoveSts(i)==2)||(MoveSts(i)==3))))
                    if (Classfication(i)==1)||(Classfication(i)==2)||(Classfication(i)==3)||(Classfication(i)==9)
                        if ((Range(i)<=TarLimS0Dx)&&(MoveSts(i)==1))||((Range(i)<=TarLimDx)&&((MoveSts(i)==2)||(MoveSts(i)==3)))
                            if (plaus(i)>=0.4)||((wCutIn(i)>0.7)&&(spw(i)>=0.8))||((spw(i)>0.95)&&(Range(i)<1.5*vRef))
                                if Range(i)<P0Range
                                    P0ID = uint8(i);
                                    P0Range = Range(i);
                                end
                            else
                                if spwLeft(i)>0.2
                                    if Range(i)<P2Range
                                        P2ID = uint8(i);
                                        P2Range = Range(i);
                                    end
                                end
                                if spwRight(i)>0.2
                                    if Range(i)<P3Range
                                        P3ID = uint8(i);
                                        P3Range = Range(i);
                                    end
                                end
                            end
                        end
                    end
                end
            end           
        end
    end
end

if (P0ID>0)&&(P0ID<100)
    TargetExist = true;
    P0Range = Range(P0ID);
    P0Vr = Vr(P0ID);
    P0ArG = ArG(P0ID);
    P0Dx = Dx(P0ID);
    P0Dy = Dy(P0ID);
    if wCutIn(P0ID)>0.6
       TargetCutIn_b = true;
    end
    P0Dyc = Dyc(P0ID);
    P0Vyc = Vyc(P0ID);
else
    if P0ID>100
        TargetExist = true;
        P0Range = ReRange;
        P0Vr = ReVx;
        P0ArG = ReArG;
        P0Dx = ReDx;
        P0Dy = ReDy;
        TargetCutIn_b = ReCutIn_b;
        P0Dyc = ReDyc;
        P0Vyc = ReVyc;
    end
end
if P2ID>0
    P2Range = Range(P2ID);
    P2Vr = Vr(P2ID);
    P2ArG = ArG(P2ID);
    P2Dx = Dx(P2ID);
    P2Dy = Dy(P2ID);
end
if P3ID>0
    P3Range = Range(P3ID);
    P3Vr = Vr(P3ID);
    P3ArG = ArG(P3ID);
    P3Dx = Dx(P3ID);
    P3Dy = Dy(P3ID);
end
end

== matlab function Noa_Nofusion_angle/TOS2/Subsystem1/ACCOSM/HWA_Task100ms1/TimeCalc ==
  data: SameTarget input boolean size=1; TargetID input uint8 size=1; tSameHandleTK1 input single size=1; tSameHandleT output single size=1
function tSameHandleT = TimeCalc(SameTarget,TargetID,tSameHandleTK1)

if TargetID~=0
    if SameTarget==true
        tSameHandleT = min(tSameHandleTK1 + single(0.1),single(1800));
    else
        tSameHandleT = single(0);
    end
else
    tSameHandleT = single(0);
end
